simulink model "untitled1"  (R2013a)
settings: Solver=ode45  StartTime=0.0  StopTime=10.0  RelTol=1e-3
libraries: dspxfrm3 x1
settings Model: Creator=hp  LastModifiedBy=hp

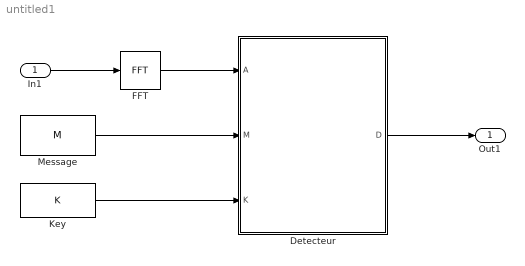
== system untitled1 ==
  In1 : Inport
  Detecteur : MATLAB Function  TreatAsAtomicUnit=on
  FFT : dspxfrm3/FFT  CompMethod=Table lookup  TableOpt=NEW  TableOptActive=Speed  BitRevOrder=off  InheritFFTLength=on  FFTLength=64  RowConvenienceOn=on  FFTImplementation=Auto  SkipNorm=off  firstCoeffDataTypeStr=Inherit: Same word length as input  firstCoeffLastDataTypeStr=Inherit: Same word length as input  outputMin=[]  outputMax=[]  roundingMode=Floor  overflowMode=off
  Key : FromWorkspace  VariableName=K  SampleTime=0
  Message : FromWorkspace  VariableName=M  SampleTime=0
  Out1 : Outport
  wires:
  In1/1 -> FFT/1
  FFT/1 -> Detecteur/1(A)
  Message/1 -> Detecteur/2(M)
  Key/1 -> Detecteur/3(K)
  Detecteur/1(D) -> Out1/1

== matlab function untitled1/Detecteur ==
  data: A input; D output; M input; K input
function D = fcn(A,M,K)
%#codegen

D = u;
